simulink library "LateralControl_fcns_lib"  (R2018b)
settings: Solver=ode45  StartTime=0.0  StopTime=10.0  RelTol=1e-3  EnableMultiTasking=on
values from neighbouring files (symbols this model uses):
  c_BIT0 = 1.0    [LCK_LogicPara.sldd]
  c_BIT1 = 2.0    [LCK_LogicPara.sldd]
  c_BIT10 = 1024.0    [LCK_LogicPara.sldd]
  c_BIT11 = 2048.0    [LCK_LogicPara.sldd]
  c_BIT12 = 4096.0    [LCK_LogicPara.sldd]
  c_BIT13 = 8192.0    [LCK_LogicPara.sldd]
  c_BIT14 = 16384.0    [LCK_LogicPara.sldd]
  c_BIT15 = 32768.0    [LCK_LogicPara.sldd]
  c_BIT2 = 4.0    [LCK_LogicPara.sldd]
  c_BIT3 = 8.0    [LCK_LogicPara.sldd]
  c_BIT4 = 16.0    [LCK_LogicPara.sldd]
  c_BIT5 = 32.0    [LCK_LogicPara.sldd]
  c_BIT6 = 64.0    [LCK_LogicPara.sldd]
  c_BIT7 = 128.0    [LCK_LogicPara.sldd]
  c_BIT8 = 256.0    [LCK_LogicPara.sldd]
  c_BIT9 = 512.0    [LCK_LogicPara.sldd]
  ML_TIME_MSEC = 20.0    [LCK_Macro.sldd]
undefined symbols (not defined in the file or in its folder): k_LCK_Valid_Range_Remain_Tm_s, k_SPP_clearance_FusGdr, k_SPP_clearance_RE, k_SPP_clearance_VisBarr, TJA_SP_CONF_LOW
libraries: $bdroot x4, simulink x3, tllib x1
(part 2 of 2)

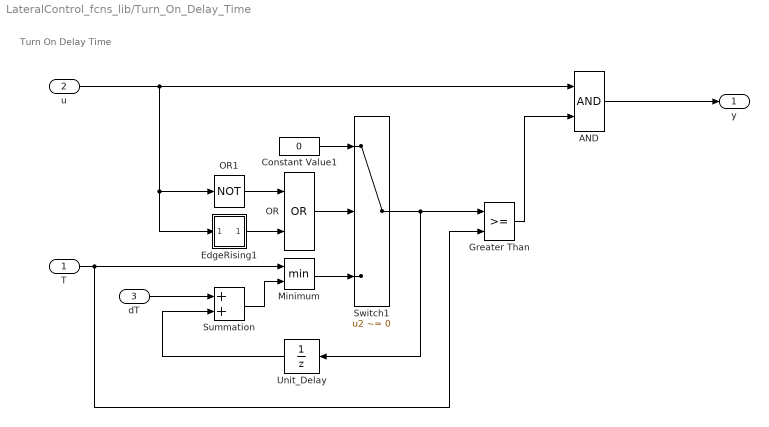
== system LateralControl_fcns_lib/Turn_On_Delay_Time ==
  note: Turn On Delay Time
  T : Inport
  u : Inport  Port=2
  dT : Inport  Port=3
  AND : Logic  OutDataTypeStr=boolean
  Constant Value1 : Constant  Value=0  OutDataTypeStr=Inherit: Inherit via back propagation
  EdgeRising1 : Subsystem  mask(EdgeRising){vinit=0}
      mask prompts: vinit "Init Codition"
      mask help: The output indicates true if the logical input value changes from false to true. Input1=Value (u).
      settings: AttributesFormatString=<Init Codition = %<vinit>>  RTWSystemCode=Inline
      mask Help: web(char(which([char(get_param(gcb,'MaskType')),'.html'])));
      mask Display:
      | color('blue');
      | plot([0.25 0.5 0.5 0.85], [0.15 0.15 0.9 0.9])
      | plot([0.38 0.5 0.62], [0.45 0.7 0.45])
  Greater Than : RelationalOperator  OutDataTypeStr=boolean  RndMeth=Nearest  InputSameDT=on
  Minimum : MinMax  Inputs=2  RndMeth=Zero  InputSameDT=on
  OR : Logic  Operator=OR  OutDataTypeStr=boolean
  OR1 : Logic  Operator=NOT  OutDataTypeStr=boolean
  Summation : Sum  RndMeth=Zero  InputSameDT=on
  Switch1 : Switch  Criteria=u2 ~= 0  Threshold=1  RndMeth=Zero  InputSameDT=on
      settings: AttributesFormatString=<%<Criteria>>
  Unit_Delay : UnitDelay  SampleTime=-1
      settings: AttributesFormatString=|
      | <init value = %<InitialCondition>>
      | <sample time = %<SampleTime>>
  y : Outport
  wires:
  u/1 -> AND/1, EdgeRising1/1(u1), OR1/1
  T/1 -> Minimum/1, Greater Than/2
  OR1/1 -> OR/1
  Minimum/1 -> Switch1/3
  dT/1 -> Summation/1
  Switch1/1 -> Unit_Delay/1, Greater Than/1
  Greater Than/1 -> AND/2
  AND/1 -> y/1
  Unit_Delay/1 -> Summation/2
  Summation/1 -> Minimum/2
  OR/1 -> Switch1/2
  Constant Value1/1 -> Switch1/1
  EdgeRising1/1(y1) -> OR/2

== system LateralControl_fcns_lib/Unit_Delay_IC ==
  n : Inport  Description=_GWMAB30P4.LKAFN.000_346_
  IC : Inport  Description=_GWMAB30P4.LKAFN.000_347_  Port=2
  Constant : Constant  Description=_GWMAB30P4.LKAFN.000_348_
  Switch : Switch  Description=_GWMAB30P4.LKAFN.000_349_  Threshold=0.5
  Unit Delay : UnitDelay  Description=_GWMAB30P4.LKAFN.000_350_  SampleTime=-1
  Unit Delay1 : UnitDelay  Description=_GWMAB30P4.LKAFN.000_351_  SampleTime=-1
  n-1 : Outport  Description=_GWMAB30P4.LKAFN.000_352_
  wires:
  n/1 -> Unit Delay1/1
  Switch/1 -> n-1/1
  IC/1 -> Switch/3
  Unit Delay/1 -> Switch/2
  Unit Delay1/1 -> Switch/1
  Constant/1 -> Unit Delay/1

== system LateralControl_fcns_lib/First_Order_Lag_Filter_LIB/Filter_Gain ==
  note: Filter Gain = T / (T + t)
      | T=> Loop time and
      | t => time constant
  note: t
  note: T
  CL_TIME : Inport  Description=_GWMAB30P4.LKAFN.000_142_
  time_constant : Inport  Description=_GWMAB30P4.LKAFN.000_143_  Port=2
  Product1 : Product  Description=_GWMAB30P4.LKAFN.000_144_  Inputs=*/
  Sum2 : Sum  Description=_GWMAB30P4.LKAFN.000_145_  OutDataTypeStr=Inherit: Same as first input
  Gain : Outport  Description=_GWMAB30P4.LKAFN.000_146_
  wires:
  time_constant/1 -> Sum2/2
  CL_TIME/1 -> Product1/1, Sum2/1
  Product1/1 -> Gain/1
  Sum2/1 -> Product1/2

== system LateralControl_fcns_lib/Turn_Off_Delay_Time/EdgeFalling1 ==
  u : Inport  OutDataTypeStr=boolean
  AND : Logic  OutDataTypeStr=boolean
  OR1 : Logic  Operator=NOT  OutDataTypeStr=boolean
  Unit_Delay : UnitDelay  InitialCondition=vinit  SampleTime=-1
      settings: AttributesFormatString=|
      | <init value = %<InitialCondition>>
      | <sample time = %<SampleTime>>
  y : Outport  OutDataTypeStr=boolean
  wires:
  OR1/1 -> AND/1
  Unit_Delay/1 -> AND/2
  AND/1 -> y/1
  u/1 -> Unit_Delay/1, OR1/1

== system LateralControl_fcns_lib/Turn_On_Delay_Time/EdgeRising1 ==
  u1 : Inport  OutDataTypeStr=boolean
  AND : Logic  OutDataTypeStr=boolean
  OR1 : Logic  Operator=NOT  OutDataTypeStr=boolean
  Unit_Delay : UnitDelay  InitialCondition=vinit  SampleTime=-1
      settings: AttributesFormatString=|
      | <init value = %<InitialCondition>>
      | <sample time = %<SampleTime>>
  y1 : Outport  OutDataTypeStr=boolean
  wires:
  OR1/1 -> AND/2
  Unit_Delay/1 -> OR1/1
  AND/1 -> y1/1
  u1/1 -> Unit_Delay/1, AND/1

== stateflow chart LateralControl_fcns_lib/Delay_Trig/Delay_Trig ==
  settings: description=|
      | _GACA26P4.LCKFN.111_5_
      | $TL$ name=$C_$O; type=Bool; class=default; $TL$
  state OFF
    en: Delay_Trig =0;
    duration= 0;
    settings: description=_GWMH9P5.LCKFN.111_2_
  state ON
    en: Delay_Trig = 0;
    duration=duration+ML_TIME_SEC;
    du:duration=duration+ML_TIME_SEC;
    settings: description=_GWMH9P5.LCKFN.111_3_
  state Trig
    en: Delay_Trig = 1;
    settings: description=_GWMH9P5.LCKFN.111_4_
  (default) -> OFF
  OFF -> ON : [(Input)]
  ON -> OFF [order 2] : [!Input]
  Trig -> OFF : [!Input]
  ON -> Trig [order 1] : [(Input) && (duration>= Delay_Trig_Time)]
  data: Input input; Delay_Trig_Time input; ML_TIME_SEC parameter single; Delay_Trig output single; duration local single
  data Input settings: description=_GWMH9P5.LCKFN.111_7_
  data Delay_Trig_Time settings: description=_GWMH9P5.LCKFN.111_8_
  data ML_TIME_SEC settings: description=_GWMAB30P3.LCKFN.111_1_$TL$ name=$O; type=Float32; class=EXTERN_MACRO; $TL$
  data Delay_Trig settings: description=_GWMH9P5.LCKFN.111_9_
  data duration settings: description=_GWMAB30P3.LCKFN.111_3_$TL$ name=$C_$O; type=Float32; class=default; $TL$

== stateflow chart LateralControl_fcns_lib/Signal_Sustain/Sustain_wo_reset ==
  settings: description=_GWMH9P4.LKAFN.111_8_
  state Hold
    en:sustain_value = input;
    du:i=i+ML_TIME_MSEC;
    settings: description=_GWMH9P4.LKAFN.111_35_
  state Standby
    en:
    i=0;
    du:
    sustain_value = 0;
    settings: description=_GWMH9P4.LKAFN.111_36_
  (default) -> Standby
  Standby -> Hold : [input]
  Hold -> Hold [order 1] : [input]
      | {i=0;}
  Hold -> Standby [order 2] : [(i>= sustain_time) && (!input)]
  data: input input; sustain_time input; sustain_value output double; ML_TIME_MSEC parameter; i local double
  data input settings: description=_GWMH9P4.LKAFN.111_71_
  data sustain_time settings: description=_GWMH9P4.LKAFN.111_72_
  data sustain_value settings: description=_GWMAB30P4.LKAFN.111_83_
  data ML_TIME_MSEC settings: description=_GWMAB30P4.LKAFN.111_84_
  data i settings: description=_GWMAB30P4.LKAFN.111_85_

== stateflow chart LateralControl_fcns_lib/Trigger Hold Counter/Trigger Hold ==
  settings: description=_GWMH9P5.LCK.111_13_
  (default) -> (junction 11)
  (junction 11) -> (junction 13) [order 1] : [(Trigger==1)]...
      | {count = 0;}
  (junction 11) -> (junction 14) [order 2]
  (junction 13) -> (junction 17)
  (junction 14) -> (junction 17) [order 1] : [(count<= hold_time)&&(count>0)]
  (junction 14) -> (junction 15) [order 2] : {Out = 0;}
  (junction 17) -> (junction 16) : {
      | Out = 1;...
      | count = count + ML_TIME_MSEC;
      | }
  (junction 15) -> (junction 16)
  (junction 16) -> (junction 25)
  data: Trigger input [0..1]; hold_time input; Out output boolean [0..1]; count output single; ML_TIME_MSEC parameter single
  data Trigger settings: description=_GWMH9P5.LCK.111_116_
  data hold_time settings: description=_GWMH9P5.LCK.111_117_
  data Out settings: description=|
      | _GACA26P4.LCK.111_66_
      | $TL$ type=Bool; date=20190416T145812; $TL$
  data count settings: description=|
      | _GACA26P4.LCK.111_67_
      | $TL$ type=Float32; date=20190416T145816; $TL$
  data ML_TIME_MSEC settings: description=|
      | _GACA26P4.LCK.111_68_
      | $TL$ name=$O; type=ESR_Typedefs/unsigned8_T; class=EXTERN_MACRO; date=20190416T150613; $TL$

== stateflow chart LateralControl_fcns_lib/Delay_Trig_Cnt/Delay_Trig ==
  settings: description=_GWMAB30P4.LKAFN.111_51_
  state OFF
    en: Delay_Trig =0;
    count= 0;
    settings: description=_GWMH9P4.LKAFN.111_17_
  state ON
    en: Delay_Trig = 0;
    count++;
    du:count++;
    settings: description=_GWMH9P4.LKAFN.111_18_
  state Trig
    en: Delay_Trig = 1;
    settings: description=_GWMH9P4.LKAFN.111_19_
  (default) -> OFF
  OFF -> ON : [(Input)]
  ON -> OFF [order 2] : [!Input]
  Trig -> OFF : [!Input]
  ON -> Trig [order 1] : [(Input) && (count>= Delay_Trig_count)]
  data: Input input; Delay_Trig_count input; count local double; Delay_Trig output
  data Input settings: description=_GWMH9P4.LKAFN.111_50_
  data Delay_Trig_count settings: description=_GWMH9P4.LKAFN.111_51_
  data count settings: description=_GWMAB30P4.LKAFN.111_50_
  data Delay_Trig settings: description=_GWMH9P4.LKAFN.111_52_

== stateflow chart LateralControl_fcns_lib/CountTrig/CountTrig ==
  settings: description=_GWMH9P5.LCKFN.111_1_
  (default) -> (junction 11)
  (junction 11) -> (junction 13) [order 1] : [(Trigger==1)]...
      | { count_enable=1;}
  (junction 11) -> (junction 15) [order 2] : {Out = 0;count_enable=0;count=0;}
  (junction 13) -> (junction 17) : {
      | count = count + ML_TIME_MSEC;
      | }
  (junction 17) -> (junction 31) [order 1] : [count== CountTrig_time&& count_enable==1]...
      | {Out=1;}
  (junction 31) -> (junction 16)
  (junction 17) -> (junction 16) [order 2] : {
      | Out=0;
      | }
  (junction 15) -> (junction 16)
  (junction 16) -> (junction 25)
  data: Trigger input double [0..1]; CountTrig_time input double; Out output double [0..1]; count local double; ML_TIME_MSEC parameter double; count_enable local double
  data Trigger settings: description=_GWMH9P5.LCKFN.111_5_
  data CountTrig_time settings: description=_GWMH9P5.LCKFN.111_6_
  data Out settings: description=|
      | _GWMH9P4.LCKFN.111_9_
      | $TL$ type=Bool; $TL$
  data count settings: description=|
      | _GWMH9P4.LCKFN.111_5_
      | $TL$ type=UInt32; $TL$
  data ML_TIME_MSEC settings: description=|
      | _GWMH9P4.LCKFN.111_10_
      | $TL$ name=$O; type=ESR_Typedefs/unsigned8_T; class=EXTERN_MACRO; $TL$
  data count_enable settings: description=|
      | _GWMH9P4.LCKFN.111_6_
      | $TL$ type=Bool; $TL$

== stateflow chart LateralControl_fcns_lib/Signal_Sustain_With_Clear/signal_sustain ==
  settings: description=_GWMH9P4.LKAFN.111_6_
  note: ML_TIME_MSEC = 10ms
  state Standby
    en:
    i = 0;
    du:
    sustain_value = 0;
    settings: description=_GWMH9P4.LKAFN.111_31_
  state Hold
    en: sustain_value = input;
    du:i = i + ML_TIME_MSEC;
    settings: description=_GWMH9P4.LKAFN.111_30_
  (default) -> Standby
  Standby -> Hold : [input && (!clear)]
  Hold -> Hold [order 1] : [(input) && (i < sustain_time) && (!clear)]
      | {i = 0;}
  Hold -> Standby [order 2] : [(i >= sustain_time) || (clear)]
  data: input input; i local single; ML_TIME_MSEC parameter single; sustain_value output single; sustain_time input; clear input
  data input settings: description=_GWMH9P4.LKAFN.111_65_
  data i settings: description=_GWMAB30P4.LKAFN.111_70_
  data ML_TIME_MSEC settings: description=_GWMAB30P4.LKAFN.111_71_
  data sustain_value settings: description=_GWMAB30P4.LKAFN.111_72_
  data sustain_time settings: description=_GWMH9P4.LKAFN.111_66_
  data clear settings: description=_GWMH9P4.LKAFN.111_67_

== stateflow chart LateralControl_fcns_lib/CR_inhibit/CR_inhibit ==
  settings: description=_GWMH9P4.LKAFN.111_1_
  note: ML_TIME_MSEC = 10ms
  state Input_Standby
    en:
    input_value = 0;
    i = 0;
    du:
    warn_output = 0;
    settings: description=_GWMH9P4.LKAFN.111_14_
  state WaitPeriod
    en:
    i = i + ML_TIME_MSEC;
    du:
    warn_output = 0;
    i = i + ML_TIME_MSEC;
    settings: description=_GWMH9P4.LKAFN.111_16_
  state Output
    du:
    warn_output =1;
    i = 0;
    settings: description=_GWMH9P4.LKAFN.111_15_
  (default) -> Input_Standby
  Input_Standby -> WaitPeriod : [current_input >k_CR_Threshold ]
      | {input_value = current_input;}
  WaitPeriod -> Input_Standby [order 2] : [current_input < k_CR_Threshold &&...
      |  i < k_mantian_msec ]
  Output -> Input_Standby : [current_input < k_CR_Threshold]
  WaitPeriod -> Output [order 1] : [ current_input > k_CR_Threshold &&...
      | i >= k_mantian_msec ]
  data: current_input input; i local single; ML_TIME_MSEC parameter single; warn_output output single; input_value local single; k_mantian_msec input; k_CR_Threshold input
  data current_input settings: description=_GWMH9P4.LKAFN.111_47_
  data i settings: description=_GWMAB30P4.LKAFN.111_42_
  data ML_TIME_MSEC settings: description=_GWMAB30P4.LKAFN.111_43_
  data warn_output settings: description=_GWMAB30P4.LKAFN.111_44_
  data input_value settings: description=_GWMAB30P4.LKAFN.111_45_
  data k_mantian_msec settings: description=_GWMH9P4.LKAFN.111_48_
  data k_CR_Threshold settings: description=_GWMH9P4.LKAFN.111_49_
